simulink subsystem "Fault_eSPAARO5"  (R2025a)
settings: Solver=VariableStepAuto  StartTime=0.0  StopTime=10.0  RelTol=1e-3
libraries: px4Utilslib x5
settings Model: Creator=gurt1  LastModifiedBy=gurt1

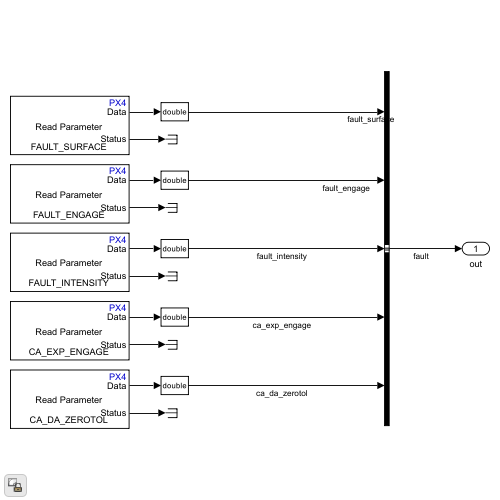
[thumbnail: Simulink's stored preview of the top-level diagram]
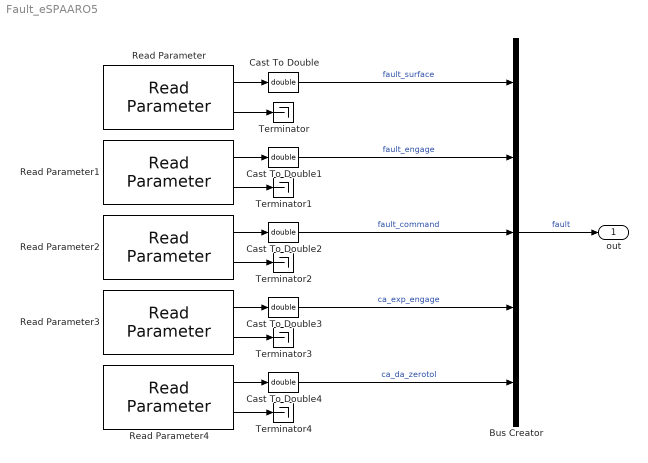
== system Fault_eSPAARO5 ==
  Bus Creator : BusCreator  Inputs=5
  Cast To Double{,1..4} (5 alike) : DataTypeConversion  OutDataTypeStr=double  SaturateOnIntegerOverflow=off  RndMeth=Floor
  Read Parameter : px4Utilslib/Read Parameter  ParameterName=FAULT_SURFACE  DataType=FLOAT  SampleTime=-1
  Read Parameter1 : px4Utilslib/Read Parameter  ParameterName=FAULT_ENGAGE  DataType=FLOAT  SampleTime=-1
  Read Parameter2 : px4Utilslib/Read Parameter  ParameterName=FAULT_COMMAND  DataType=FLOAT  SampleTime=-1
  Read Parameter3 : px4Utilslib/Read Parameter  ParameterName=CA_EXP_ENGAGE  DataType=FLOAT  SampleTime=-1
  Read Parameter4 : px4Utilslib/Read Parameter  ParameterName=CA_DA_ZEROTOL  DataType=FLOAT  SampleTime=-1
  Terminator{,1..4} (5 alike) : Terminator
  out : Outport
  wires:
  Read Parameter/2 -> Terminator/1
  Read Parameter/1 -> Cast To Double/1
  Cast To Double/1 -> Bus Creator/1  "fault_surface"
  Read Parameter1/1 -> Cast To Double1/1
  Read Parameter1/2 -> Terminator1/1
  Cast To Double1/1 -> Bus Creator/2  "fault_engage"
  Bus Creator/1 -> out/1  "fault"
  Read Parameter2/1 -> Cast To Double2/1
  Read Parameter2/2 -> Terminator2/1
  Cast To Double2/1 -> Bus Creator/3  "fault_command"
  Read Parameter3/2 -> Terminator3/1
  Read Parameter3/1 -> Cast To Double3/1
  Cast To Double3/1 -> Bus Creator/4  "ca_exp_engage"
  Read Parameter4/1 -> Cast To Double4/1
  Cast To Double4/1 -> Bus Creator/5  "ca_da_zerotol"
  Read Parameter4/2 -> Terminator4/1
